simulink model "Van3"  (R2024b)
settings: Solver=ode3  StartTime=0.0  StopTime=10  FixedStep=0.001  RelTol=1e-3
Description:
  | 自适应控制
settings Model: PacingRate=1000  Creator=繁星  LastModifiedBy=14422
settings SolverCC: ShapePreserveControl=EnableAll  ZeroCrossAlgorithm=Adaptive  EnableFixedStepZeroCrossing=on
settings DataIOCC: ReturnWorkspaceOutputs=off
settings OptimizationCC: ReuseModelBlockBuffer=off
settings ModelReferenceCC: EnableRefExpFcnMdlSchedulingChecks=on
settings RTWCC: GPUComputeCapability=3.5

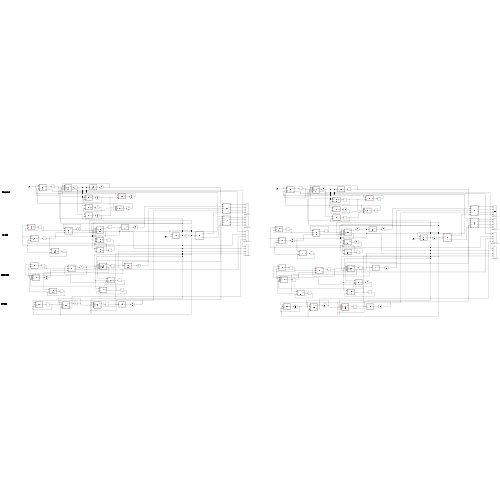
[thumbnail: Simulink's stored preview of the top-level diagram]
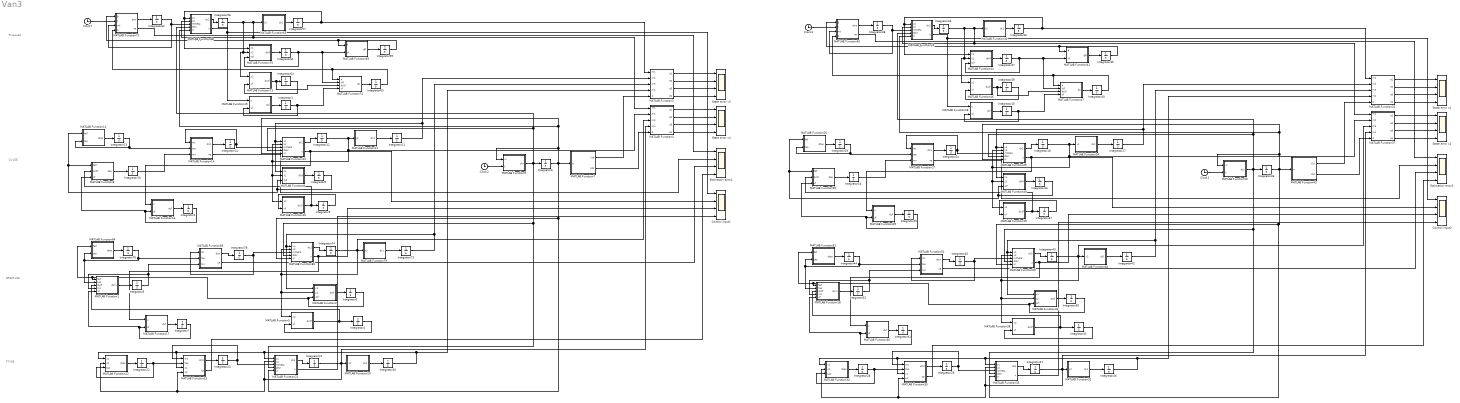
== system Van3 ==
  note: DREM-LSE
  note: CL-LSE
  note: FT-lSE
  note: Proposed
  Clock{1..3,7} (4 alike) : Clock
  Control input1 : Scope  NumInputPorts=4
  Control input2 : Scope  NumInputPorts=4
  Estimation error1 : Scope  NumInputPorts=4
  Estimation error2 : Scope  NumInputPorts=4
  Integrator{1..4,7..9,12,15,21,25,30,37..38,40..41,46,58,61..62,64..65,74} (23 alike) : Integrator
  Integrator{5,10,16,32} (4 alike) : Integrator  InitialCondition=[0;0;0]
  Integrator{11,20,57,73} (4 alike) : Integrator  InitialCondition=1
  Integrator{13,19,22,44,76} (5 alike) : Integrator  InitialCondition=1000*eye(3)
  Integrator{14,23..24,29,45,78} (6 alike) : Integrator  InitialCondition=[0.5;-1;1]*0
  Integrator{17,26,33,42} (4 alike) : Integrator  InitialCondition=0.8
  Integrator{18,27,34,43} (4 alike) : Integrator  InitialCondition=-0.5
  Integrator28 : Integrator  InitialCondition=1000*eye(3)  UpperSaturationLimit=1000  LowerSaturationLimit=0
  Integrator31 : Integrator  InitialCondition=-5
  Integrator35 : Integrator  InitialCondition=[1 0 0;0 1 0;0 0 1]*1e-7
  Integrator36 : Integrator  InitialCondition=[1;0]
  Integrator39 : Integrator  InitialCondition=-5
  Integrator47 : Integrator  InitialCondition=-5
  Integrator59 : Integrator  InitialCondition=[1 0 0;0 1 0;0 0 1]*1e-7
  Integrator6 : Integrator  InitialCondition=[1;0]
  MATLAB Function1 : MATLAB Function  TreatAsAtomicUnit=on
  MATLAB Function10 : MATLAB Function  TreatAsAtomicUnit=on
  MATLAB Function11 : MATLAB Function  TreatAsAtomicUnit=on
  MATLAB Function12 : MATLAB Function  TreatAsAtomicUnit=on
  MATLAB Function13 : MATLAB Function  TreatAsAtomicUnit=on
  MATLAB Function14 : MATLAB Function  TreatAsAtomicUnit=on
  MATLAB Function15 : MATLAB Function  TreatAsAtomicUnit=on
  MATLAB Function16 : MATLAB Function  TreatAsAtomicUnit=on
  MATLAB Function17 : MATLAB Function  TreatAsAtomicUnit=on
  MATLAB Function18 : MATLAB Function  TreatAsAtomicUnit=on
  MATLAB Function19 : MATLAB Function  TreatAsAtomicUnit=on
  MATLAB Function2 : MATLAB Function  TreatAsAtomicUnit=on
  MATLAB Function20 : MATLAB Function  TreatAsAtomicUnit=on
  MATLAB Function21 : MATLAB Function  TreatAsAtomicUnit=on
  MATLAB Function22 : MATLAB Function  TreatAsAtomicUnit=on
  MATLAB Function23 : MATLAB Function  TreatAsAtomicUnit=on
  MATLAB Function24 : MATLAB Function  TreatAsAtomicUnit=on
  MATLAB Function25 : MATLAB Function  TreatAsAtomicUnit=on
  MATLAB Function26 : MATLAB Function  TreatAsAtomicUnit=on
  MATLAB Function27 : MATLAB Function  TreatAsAtomicUnit=on
  MATLAB Function28 : MATLAB Function  TreatAsAtomicUnit=on
  MATLAB Function29 : MATLAB Function  TreatAsAtomicUnit=on
  MATLAB Function3 : MATLAB Function  TreatAsAtomicUnit=on
  MATLAB Function30 : MATLAB Function  TreatAsAtomicUnit=on
  MATLAB Function31 : MATLAB Function  TreatAsAtomicUnit=on
  MATLAB Function32 : MATLAB Function  TreatAsAtomicUnit=on
  MATLAB Function33 : MATLAB Function  TreatAsAtomicUnit=on
  MATLAB Function34 : MATLAB Function  TreatAsAtomicUnit=on
  MATLAB Function35 : MATLAB Function  TreatAsAtomicUnit=on
  MATLAB Function36 : MATLAB Function  TreatAsAtomicUnit=on
  MATLAB Function37 : MATLAB Function  TreatAsAtomicUnit=on
  MATLAB Function38 : MATLAB Function  TreatAsAtomicUnit=on
  MATLAB Function39 : MATLAB Function  TreatAsAtomicUnit=on
  MATLAB Function4 : MATLAB Function  TreatAsAtomicUnit=on
  MATLAB Function40 : MATLAB Function  TreatAsAtomicUnit=on
  MATLAB Function41 : MATLAB Function  TreatAsAtomicUnit=on
  MATLAB Function42 : MATLAB Function  TreatAsAtomicUnit=on
  MATLAB Function43 : MATLAB Function  TreatAsAtomicUnit=on
  MATLAB Function44 : MATLAB Function  TreatAsAtomicUnit=on
  MATLAB Function45 : MATLAB Function  TreatAsAtomicUnit=on
  MATLAB Function46 : MATLAB Function  TreatAsAtomicUnit=on
  MATLAB Function47 : MATLAB Function  TreatAsAtomicUnit=on
  MATLAB Function48 : MATLAB Function  TreatAsAtomicUnit=on
  MATLAB Function49 : MATLAB Function  TreatAsAtomicUnit=on
  MATLAB Function5 : MATLAB Function  TreatAsAtomicUnit=on
  MATLAB Function50 : MATLAB Function  TreatAsAtomicUnit=on
  MATLAB Function51 : MATLAB Function  TreatAsAtomicUnit=on
  MATLAB Function52 : MATLAB Function  TreatAsAtomicUnit=on
  MATLAB Function53 : MATLAB Function  TreatAsAtomicUnit=on
  MATLAB Function6 : MATLAB Function  TreatAsAtomicUnit=on
  MATLAB Function65 : MATLAB Function  TreatAsAtomicUnit=on
  MATLAB Function68 : MATLAB Function  TreatAsAtomicUnit=on
  MATLAB Function69 : MATLAB Function  TreatAsAtomicUnit=on
  MATLAB Function7 : MATLAB Function  TreatAsAtomicUnit=on
  MATLAB Function70 : MATLAB Function  TreatAsAtomicUnit=on
  MATLAB Function72 : MATLAB Function  TreatAsAtomicUnit=on
  MATLAB Function73 : MATLAB Function  TreatAsAtomicUnit=on
  MATLAB Function74 : MATLAB Function  TreatAsAtomicUnit=on
  MATLAB Function79 : MATLAB Function  TreatAsAtomicUnit=on
  MATLAB Function8 : MATLAB Function  TreatAsAtomicUnit=on
  MATLAB Function80 : MATLAB Function  TreatAsAtomicUnit=on
  MATLAB Function84 : MATLAB Function  TreatAsAtomicUnit=on
  MATLAB Function85 : MATLAB Function  TreatAsAtomicUnit=on
  MATLAB Function9 : MATLAB Function  TreatAsAtomicUnit=on
  State error x{1..4} (4 alike) : Scope  NumInputPorts=4
  wires:
  MATLAB Function73/1(dx2f) -> MATLAB Function74/3(dx2f), Integrator64/1
  MATLAB Function80/1(dx2) -> Integrator74/1
  MATLAB Function79/1(dx1) -> Integrator73/1
  MATLAB Function84/1(dtao) -> Integrator76/1
  Integrator78/1 -> MATLAB Function85/1(mt), MATLAB Function80/3(mtheta)
  Integrator62/1 -> MATLAB Function68/3(mtheta), MATLAB Function72/3(mt)
  Integrator76/1 -> MATLAB Function1/2(tao), MATLAB Function84/2(tao), MATLAB Function85/2(tao)
  MATLAB Function85/1(dmt) -> Integrator78/1
  MATLAB Function69/1(dff) -> Integrator59/1
  Integrator59/1 -> MATLAB Function72/1(B), MATLAB Function69/1(ff)
  MATLAB Function68/1(dx2) -> Integrator58/1
  MATLAB Function70/1(dWf) -> Integrator61/1
  Integrator61/1 -> MATLAB Function70/3(Wf), MATLAB Function74/2(Wf), MATLAB Function69/2(yf)
  MATLAB Function74/1(dA) -> Integrator65/1
  Integrator65/1 -> MATLAB Function72/4(A), MATLAB Function74/1(A)
  MATLAB Function65/1(dx1) -> Integrator57/1
  Integrator64/1 -> MATLAB Function73/2(xf)
  MATLAB Function72/1(dmt) -> Integrator62/1
  Clock7/1 -> MATLAB Function72/2(t)
  Integrator58/1 -> MATLAB Function68/2(x2), MATLAB Function4/1(m1), MATLAB Function65/1(x2), MATLAB Function70/2(x2), MATLAB Function73/1(x2)
  MATLAB Function3/1(dWf) -> Integrator3/1
  Integrator4/1 -> MATLAB Function5/2(xf)
  MATLAB Function5/1(dx2f) -> MATLAB Function1/3(dx2f), Integrator4/1
  Integrator3/1 -> MATLAB Function84/1(faif), MATLAB Function1/1(faif), MATLAB Function3/3(Wf)
  MATLAB Function1/1(dmn) -> Integrator5/1
  Integrator5/1 -> MATLAB Function1/4(mn), MATLAB Function85/3(mn)
  Integrator74/1 -> MATLAB Function4/3(m3), MATLAB Function5/1(x2), MATLAB Function3/2(x2), MATLAB Function80/2(x2), MATLAB Function79/1(x2)
  Integrator9/1 -> MATLAB Function10/2(xf)
  MATLAB Function8/1(dWf) -> Integrator8/1
  MATLAB Function6/1(dep) -> Integrator10/1
  MATLAB Function10/1(dx2f) -> Integrator9/1, MATLAB Function6/2(dx2f)
  Integrator14/1 -> MATLAB Function14/1(mt), MATLAB Function12/3(mtheta)
  MATLAB Function11/1(dx1) -> Integrator11/1
  MATLAB Function14/1(dmt) -> Integrator14/1
  Integrator12/1 -> MATLAB Function10/1(x2), MATLAB Function8/2(x2), MATLAB Function12/2(x2), MATLAB Function4/2(m2), MATLAB Function11/1(x2)
  MATLAB Function13/1(dtao) -> Integrator13/1
  Integrator8/1 -> MATLAB Function8/3(Wf), MATLAB Function13/1(faif), MATLAB Function6/1(faif)
  MATLAB Function12/1(dx2) -> Integrator12/1
  Integrator10/1 -> MATLAB Function14/3(mn)
  Integrator22/1 -> MATLAB Function22/3(tao), MATLAB Function23/2(tao)
  Integrator23/1 -> MATLAB Function21/3(mtheta), MATLAB Function23/1(mt)
  MATLAB Function20/1(dx1) -> Integrator20/1
  MATLAB Function23/1(dmt) -> Integrator23/1
  Integrator21/1 -> MATLAB Function4/4(m4), MATLAB Function20/1(x2), MATLAB Function23/4(x2), MATLAB Function22/2(x2), MATLAB Function21/2(x2)
  MATLAB Function22/1(dtao) -> Integrator22/1
  MATLAB Function21/1(dx2) -> Integrator21/1
  Integrator13/1 -> MATLAB Function14/2(tao), MATLAB Function13/2(tao)
  Integrator57/1 -> MATLAB Function70/1(x1), MATLAB Function68/1(x1), MATLAB Function2/1(m1)
  Integrator11/1 -> MATLAB Function2/2(m2), MATLAB Function8/1(x1), MATLAB Function12/1(x1)
  Integrator73/1 -> MATLAB Function2/3(m3), MATLAB Function3/1(x1), MATLAB Function80/1(x1)
  Integrator20/1 -> MATLAB Function22/1(x1), MATLAB Function23/3(x1), MATLAB Function21/1(x1), MATLAB Function2/4(m4)
  MATLAB Function2/2(e2) -> State error x3/2
  MATLAB Function4/1(e1) -> State error x4/1
  MATLAB Function4/2(e2) -> State error x4/2
  MATLAB Function4/4(e4) -> State error x4/4
  MATLAB Function4/3(e3) -> State error x4/3
  MATLAB Function2/3(e3) -> State error x3/3
  MATLAB Function2/4(e4) -> State error x3/4
  MATLAB Function2/1(e1) -> State error x3/1
  Clock2/1 -> MATLAB Function9/2(t)
  Integrator6/1 -> MATLAB Function21/5(xr), MATLAB Function80/5(xr), MATLAB Function12/5(xr), MATLAB Function68/5(xr), MATLAB Function9/1(xr), MATLAB Function7/1(xr)
  MATLAB Function9/1(dxr) -> MATLAB Function80/4(ddxr), MATLAB Function21/4(ddxr), MATLAB Function12/4(ddxr), MATLAB Function68/4(ddxr), Integrator6/1
  MATLAB Function7/1(x1d) -> MATLAB Function2/5(d)
  MATLAB Function7/2(x2d) -> MATLAB Function4/5(d)
  MATLAB Function72/2(ne) -> Estimation error1/1
  MATLAB Function14/2(ne) -> Estimation error1/2
  MATLAB Function85/2(ne) -> Estimation error1/3
  MATLAB Function23/2(ne) -> Estimation error1/4
  MATLAB Function21/2(u) -> Control input1/4
  MATLAB Function80/2(u) -> MATLAB Function17/1(u), Control input1/3
  MATLAB Function12/2(u) -> MATLAB Function16/1(u), Control input1/2
  MATLAB Function68/2(u) -> MATLAB Function15/1(u), Control input1/1
  MATLAB Function15/1(duf) -> Integrator1/1
  Integrator1/1 -> MATLAB Function74/4(uf), MATLAB Function15/2(uf)
  MATLAB Function16/1(duf) -> Integrator2/1
  Integrator2/1 -> MATLAB Function6/3(uf), MATLAB Function16/2(uf)
  Integrator7/1 -> MATLAB Function1/5(uf), MATLAB Function17/2(uf)
  MATLAB Function17/1(duf) -> Integrator7/1
  MATLAB Function31/4(e4) -> State error x1/4
  MATLAB Function31/1(e1) -> State error x1/1
  MATLAB Function37/3(e3) -> State error x2/3
  MATLAB Function37/1(e1) -> State error x2/1
  MATLAB Function31/2(e2) -> State error x1/2
  Integrator15/1 -> MATLAB Function47/4(uf), MATLAB Function28/2(uf)
  MATLAB Function37/2(e2) -> State error x2/2
  MATLAB Function36/1(dWf) -> Integrator30/1
  MATLAB Function40/1(dx1) -> Integrator33/1
  MATLAB Function49/1(dWf) -> Integrator46/1
  MATLAB Function50/1(dx2) -> Integrator43/1
  Integrator32/1 -> MATLAB Function18/4(mn), MATLAB Function52/3(mn)
  MATLAB Function51/1(dtao) -> Integrator44/1
  MATLAB Function44/1(dWf) -> Integrator37/1
  Integrator19/1 -> MATLAB Function27/2(tao), MATLAB Function26/2(tao)
  Integrator28/1 -> MATLAB Function34/3(tao), MATLAB Function35/2(tao)
  Integrator37/1 -> MATLAB Function44/3(Wf), MATLAB Function47/2(Wf), MATLAB Function42/2(yf)
  MATLAB Function18/1(dmn) -> Integrator32/1
  MATLAB Function39/1(dep) -> Integrator16/1
  MATLAB Function26/1(dtao) -> Integrator19/1
  MATLAB Function35/1(dmt) -> Integrator29/1
  Clock3/1 -> MATLAB Function45/2(t)
  MATLAB Function33/1(dx2) -> Integrator27/1
  Integrator44/1 -> MATLAB Function18/2(tao), MATLAB Function51/2(tao), MATLAB Function52/2(tao)
  MATLAB Function19/1(dx2f) -> Integrator47/1, MATLAB Function39/2(dx2f)
  Integrator40/1 -> MATLAB Function45/4(A), MATLAB Function47/1(A)
  Integrator16/1 -> MATLAB Function27/3(mn)
  MATLAB Function42/1(dff) -> Integrator35/1
  MATLAB Function31/3(e3) -> State error x1/3
  Integrator24/1 -> MATLAB Function27/1(mt), MATLAB Function25/3(mtheta)
  MATLAB Function41/1(dx2) -> Integrator34/1
  Integrator34/1 -> MATLAB Function41/2(x2), MATLAB Function37/1(m1), MATLAB Function40/1(x2), MATLAB Function44/2(x2), MATLAB Function46/1(x2)
  MATLAB Function41/2(u) -> MATLAB Function28/1(u), Control input2/1
  MATLAB Function53/1(dxr) -> MATLAB Function50/4(ddxr), MATLAB Function33/4(ddxr), MATLAB Function25/4(ddxr), MATLAB Function41/4(ddxr), Integrator36/1
  Integrator36/1 -> MATLAB Function33/5(xr), MATLAB Function50/5(xr), MATLAB Function25/5(xr), MATLAB Function41/5(xr), MATLAB Function53/1(xr), MATLAB Function43/1(xr)
  Clock1/1 -> MATLAB Function53/2(t)
  Integrator26/1 -> MATLAB Function34/1(x1), MATLAB Function35/3(x1), MATLAB Function33/1(x1), MATLAB Function31/4(m4)
  Integrator17/1 -> MATLAB Function31/2(m2), MATLAB Function49/1(x1), MATLAB Function25/1(x1)
  Integrator27/1 -> MATLAB Function37/4(m4), MATLAB Function32/1(x2), MATLAB Function34/2(x2), MATLAB Function35/4(x2), MATLAB Function33/2(x2)
  MATLAB Function29/1(duf) -> Integrator25/1
  Integrator25/1 -> MATLAB Function39/3(uf), MATLAB Function29/2(uf)
  MATLAB Function52/2(ne) -> Estimation error2/3
  MATLAB Function45/2(ne) -> Estimation error2/1
  MATLAB Function30/1(duf) -> Integrator41/1
  MATLAB Function27/2(ne) -> Estimation error2/2
  Integrator41/1 -> MATLAB Function18/5(uf), MATLAB Function30/2(uf)
  Integrator33/1 -> MATLAB Function44/1(x1), MATLAB Function41/1(x1), MATLAB Function31/1(m1)
  Integrator43/1 -> MATLAB Function37/3(m3), MATLAB Function38/1(x2), MATLAB Function36/2(x2), MATLAB Function50/2(x2), MATLAB Function48/1(x2)
  MATLAB Function35/2(ne) -> Estimation error2/4
  Integrator38/1 -> MATLAB Function41/3(mtheta), MATLAB Function45/3(mt)
  MATLAB Function46/1(dx2f) -> MATLAB Function47/3(dx2f), Integrator39/1
  MATLAB Function43/2(x2d) -> MATLAB Function37/5(d)
  MATLAB Function32/1(dx1) -> Integrator26/1
  MATLAB Function28/1(duf) -> Integrator15/1
  MATLAB Function43/1(x1d) -> MATLAB Function31/5(d)
  MATLAB Function25/1(dx2) -> Integrator18/1
  MATLAB Function37/4(e4) -> State error x2/4
  Integrator42/1 -> MATLAB Function31/3(m3), MATLAB Function36/1(x1), MATLAB Function50/1(x1)
  Integrator47/1 -> MATLAB Function19/2(xf)
  Integrator29/1 -> MATLAB Function33/3(mtheta), MATLAB Function35/1(mt)
  Integrator31/1 -> MATLAB Function38/2(xf)
  Integrator35/1 -> MATLAB Function45/1(B), MATLAB Function42/1(ff)
  MATLAB Function52/1(dmt) -> Integrator45/1
  MATLAB Function27/1(dmt) -> Integrator24/1
  Integrator30/1 -> MATLAB Function51/1(faif), MATLAB Function18/1(faif), MATLAB Function36/3(Wf)
  MATLAB Function47/1(dA) -> Integrator40/1
  Integrator39/1 -> MATLAB Function46/2(xf)
  MATLAB Function38/1(dx2f) -> MATLAB Function18/3(dx2f), Integrator31/1
  Integrator45/1 -> MATLAB Function52/1(mt), MATLAB Function50/3(mtheta)
  MATLAB Function45/1(dmt) -> Integrator38/1
  MATLAB Function33/2(u) -> Control input2/4
  MATLAB Function48/1(dx1) -> Integrator42/1
  Integrator46/1 -> MATLAB Function49/3(Wf), MATLAB Function26/1(faif), MATLAB Function39/1(faif)
  Integrator18/1 -> MATLAB Function19/1(x2), MATLAB Function49/2(x2), MATLAB Function25/2(x2), MATLAB Function37/2(m2), MATLAB Function24/1(x2)
  MATLAB Function24/1(dx1) -> Integrator17/1
  MATLAB Function50/2(u) -> MATLAB Function30/1(u), Control input2/3
  MATLAB Function25/2(u) -> MATLAB Function29/1(u), Control input2/2
  MATLAB Function34/1(dtao) -> Integrator28/1

== matlab function Van3/MATLAB Function14 ==
  data: dmt output size=3,1; mt input; tao input; mn input; ne output
function [dmt,ne]   = fcn(mt,tao,mn)



theta=[0.5;-1;1];

Q=inv(tao)-inv(1000*eye(3));

gama=100;

ne=norm(theta-mt);
dmt=gama*tao*(mn-Q*mt);

== matlab function Van3/MATLAB Function6 ==
  data: faif input; dep output; dx2f input; uf input
function dep = fcn(faif,dx2f,uf)



dep=faif'*(dx2f-uf);

== matlab function Van3/MATLAB Function2 ==
  data: m1 input; e1 output; m2 input; m3 input; e2 output; e3 output; m4 input; e4 output; d input
function [e1,e2,e3,e4]  = fcn(m1,m2,m3,m4,d)



e1=norm(m1-d);
e2=norm(m2-d);
e3=norm(m3-d);
e4=norm(m4-d);
e1=norm(m1-d);
e2=norm(m2-d);
e3=norm(m3-d);
e4=norm(m4-d);

== matlab function Van3/MATLAB Function8 ==
  data: x1 input; dWf output; x2 input; Wf input
function dWf  = fcn(x1,x2,Wf)

A=[-x1,x2,-x1*x1*x2];
dWf=-0.1*Wf+A;

== matlab function Van3/MATLAB Function15 ==
  data: u input; uf input; duf output
function duf  = fcn(u,uf)


duf=-0.1*uf+u;

== matlab function Van3/MATLAB Function16 ==
  data: u input; uf input; duf output
function duf  = fcn(u,uf)


duf=-0.1*uf+u;

== matlab function Van3/MATLAB Function17 ==
  data: u input; uf input; duf output
function duf  = fcn(u,uf)


duf=-0.1*uf+u;

== matlab function Van3/MATLAB Function4 ==
  data: m1 input; e1 output; m2 input; m3 input; e2 output; e3 output; m4 input; e4 output; d input
function [e1,e2,e3,e4]  = fcn(m1,m2,m3,m4,d)



e1=norm(m1-d);
e2=norm(m2-d);
e3=norm(m3-d);
e4=norm(m4-d);
e1=norm(m1-d);
e2=norm(m2-d);
e3=norm(m3-d);
e4=norm(m4-d);

== matlab function Van3/MATLAB Function18 ==
  data: faif input; dmn output; tao input; dx2f input; mn input; uf input
function dmn = fcn(faif,tao,dx2f,mn,uf)



dmn=tao*faif'*(dx2f-uf-faif*mn);

== matlab function Van3/MATLAB Function19 ==
  data: x2 input; xf input; dx2f output
function dx2f  = fcn(x2,xf)


dx2f=-0.1*xf+x2;

== matlab function Van3/MATLAB Function20 ==
  data: x2 input; dx1 output
function dx1 = fcn(x2)
dx1=x2;

== matlab function Van3/MATLAB Function21 ==
  data: x1 input; x2 input; dx2 output; mtheta input; ddxr input; xr input; u output
function [dx2,u] = fcn(x1,x2,mtheta,ddxr,xr)


%unknown parameter vector
theta=[0.5;-1;1];

x=[x1;x2];


u=ddxr(2)-[4 4]*(x-xr)-[-x1,x2,-x1*x1*x2]*mtheta;


dx2=[-x1,x2,-x1*x1*x2]*theta+u;

== matlab function Van3/MATLAB Function22 ==
  data: x1 input; x2 input; dtao output; tao input
function dtao = fcn(x1,x2,tao)


fai=[-x1,x2,-x1*x1*x2];

dtao=-tao*fai'*fai*tao;

== matlab function Van3/MATLAB Function23 ==
  data: dmt output size=3,1; mt input; ne output; tao input; x1 input; x2 input
function [dmt,ne]   = fcn(mt,tao,x1,x2)



theta=[0.5;-1;1];
fai=[-x1,x2,-x1*x1*x2];


  ne=norm(theta-mt);


dmt=tao*fai'*fai*(theta-mt);

== matlab function Van3/MATLAB Function24 ==
  data: x2 input; dx1 output
function dx1 = fcn(x2)
dx1=x2;

== matlab function Van3/MATLAB Function25 ==
  data: x1 input; x2 input; dx2 output; mtheta input; ddxr input; xr input; u output
function [dx2,u] = fcn(x1,x2,mtheta,ddxr,xr)


%unknown parameter vector
theta=[0.5;-1;1];
theta=[2;-2;3];
theta=[2;-2;3]*2;

x=[x1;x2];


u=ddxr(2)-[4 4]*(x-xr)-[-x1,x2,-x1*x1*x2]*mtheta;


dx2=[-x1,x2,-x1*x1*x2]*theta+u;

== matlab function Van3/MATLAB Function1 ==
  data: faif input; dmn output; tao input; dx2f input; mn input; uf input
function dmn = fcn(faif,tao,dx2f,mn,uf)



dmn=tao*faif'*(dx2f-uf-faif*mn);

== matlab function Van3/MATLAB Function26 ==
  data: faif input; dtao output; tao input
function dtao = fcn(faif,tao)


dtao=-tao*faif'*faif*tao;

== matlab function Van3/MATLAB Function27 ==
  data: dmt output size=3,1; mt input; tao input; mn input; ne output
function [dmt,ne]   = fcn(mt,tao,mn)



theta=[0.5;-1;1];
theta=[2;-2;3];
theta=[2;-2;3]*2;

Q=inv(tao)-inv(1000*eye(3));

gama=100;

ne=norm(theta-mt);
dmt=gama*tao*(mn-Q*mt);

== matlab function Van3/MATLAB Function28 ==
  data: u input; uf input; duf output
function duf  = fcn(u,uf)


duf=-0.1*uf+u;

== matlab function Van3/MATLAB Function29 ==
  data: u input; uf input; duf output
function duf  = fcn(u,uf)


duf=-0.1*uf+u;

== matlab function Van3/MATLAB Function30 ==
  data: u input; uf input; duf output
function duf  = fcn(u,uf)


duf=-0.1*uf+u;

== matlab function Van3/MATLAB Function31 ==
  data: m1 input; e1 output; m2 input; m3 input; e2 output; e3 output; m4 input; e4 output; d input
function [e1,e2,e3,e4]  = fcn(m1,m2,m3,m4,d)



e1=norm(m1-d);
e2=norm(m2-d);
e3=norm(m3-d);
e4=norm(m4-d);

== matlab function Van3/MATLAB Function32 ==
  data: x2 input; dx1 output
function dx1 = fcn(x2)
dx1=x2;

== matlab function Van3/MATLAB Function33 ==
  data: x1 input; x2 input; dx2 output; mtheta input; ddxr input; xr input; u output
function [dx2,u] = fcn(x1,x2,mtheta,ddxr,xr)


%unknown parameter vector
theta=[0.5;-1;1];
theta=[2;-2;3];
theta=[2;-2;3]*2;

x=[x1;x2];


u=ddxr(2)-[4 4]*(x-xr)-[-x1,x2,-x1*x1*x2]*mtheta;


dx2=[-x1,x2,-x1*x1*x2]*theta+u;

== matlab function Van3/MATLAB Function34 ==
  data: x1 input; x2 input; dtao output; tao input
function dtao = fcn(x1,x2,tao)


fai=[-x1,x2,-x1*x1*x2];

dtao=-tao*fai'*fai*tao;

== matlab function Van3/MATLAB Function35 ==
  data: dmt output size=3,1; mt input; ne output; tao input; x1 input; x2 input
function [dmt,ne]   = fcn(mt,tao,x1,x2)



theta=[0.5;-1;1];
theta=[2;-2;3];
theta=[2;-2;3]*2;
fai=[-x1,x2,-x1*x1*x2];


  ne=norm(theta-mt);


dmt=tao*fai'*fai*(theta-mt);

== matlab function Van3/MATLAB Function36 ==
  data: x1 input; dWf output; x2 input; Wf input
function dWf  = fcn(x1,x2,Wf)

A=[-x1,x2,-x1*x1*x2];
dWf=-0.1*Wf+A;

== matlab function Van3/MATLAB Function37 ==
  data: m1 input; e1 output; m2 input; m3 input; e2 output; e3 output; m4 input; e4 output; d input
function [e1,e2,e3,e4]  = fcn(m1,m2,m3,m4,d)



e1=norm(m1-d);
e2=norm(m2-d);
e3=norm(m3-d);
e4=norm(m4-d);

== matlab function Van3/MATLAB Function7 ==
  data: x1d output size=1; xr input double; x2d output size=1
function [x1d,x2d]  = fcn(xr)



x1d=xr(1);
x2d=xr(2);

== matlab function Van3/MATLAB Function38 ==
  data: x2 input; xf input; dx2f output
function dx2f  = fcn(x2,xf)


dx2f=-0.1*xf+x2;

== matlab function Van3/MATLAB Function39 ==
  data: faif input; dep output; dx2f input; uf input
function dep = fcn(faif,dx2f,uf)



dep=faif'*(dx2f-uf);

== matlab function Van3/MATLAB Function40 ==
  data: x2 input; dx1 output
function dx1 = fcn(x2)
dx1=x2;

== matlab function Van3/MATLAB Function41 ==
  data: x1 input; x2 input size=1; dx2 output size=1; mtheta input; ddxr input; xr input; u output
function [dx2,u] = fcn(x1,x2,mtheta,ddxr,xr)


%unknown parameter vector
theta=[0.5;-1;1];
theta=[2;-2;3]*2;

x=[x1;x2];


u=ddxr(2)-[4 4]*(x-xr)-[-x1,x2,-x1*x1*x2]*mtheta;


dx2=[-x1,x2,-x1*x1*x2]*theta+u;

== matlab function Van3/MATLAB Function42 ==
  data: ff input; dff output; yf input
function dff = fcn(ff,yf)


dff=-1*ff+yf'*yf;

== matlab function Van3/MATLAB Function43 ==
  data: x1d output size=1; xr input double; x2d output size=1
function [x1d,x2d]  = fcn(xr)



x1d=xr(1);
x2d=xr(2);

== matlab function Van3/MATLAB Function44 ==
  data: x1 input; dWf output; x2 input; Wf input
function dWf  = fcn(x1,x2,Wf)

A=[-x1,x2,-x1*x1*x2];
dWf=-0.1*Wf+A;

== matlab function Van3/MATLAB Function45 ==
  data: B input; dmt output size=3,1; t input; mt input; A input size=3,1; ne output
function [dmt,ne]    = fcn(B,t,mt,A)





theta=[0.5;-1;1];
theta=[2;-2;3]*2;
k1=1e-7;

  ne=norm(theta-mt);

 k=0.2;

ee=B\A-(1*eye(3)-k1*eye(3)*exp(-1*t)/B)*mt;

dmt=exp(abs(ee).^k).*sign(ee).*abs(ee).^(1-k)/(k*2);

== matlab function Van3/MATLAB Function3 ==
  data: x1 input; dWf output; x2 input; Wf input
function dWf  = fcn(x1,x2,Wf)

A=[-x1,x2,-x1*x1*x2];
dWf=-0.1*Wf+A;

== matlab function Van3/MATLAB Function46 ==
  data: x2 input; xf input; dx2f output
function dx2f  = fcn(x2,xf)


dx2f=-0.1*xf+x2;

== matlab function Van3/MATLAB Function47 ==
  data: A input; dA output; Wf input; dx2f input; uf input
function dA  = fcn(A,Wf,dx2f,uf)

theta=[0.5;-1;1];
dA=-1*A+Wf'*(dx2f-uf);
% dA=-1*A+Wf'*Wf*theta;

== matlab function Van3/MATLAB Function48 ==
  data: x2 input; dx1 output
function dx1 = fcn(x2)
dx1=x2;

== matlab function Van3/MATLAB Function49 ==
  data: x1 input; dWf output; x2 input; Wf input
function dWf  = fcn(x1,x2,Wf)

A=[-x1,x2,-x1*x1*x2];
dWf=-0.1*Wf+A;

== matlab function Van3/MATLAB Function50 ==
  data: x1 input; x2 input; dx2 output; mtheta input; ddxr input; xr input; u output
function [dx2,u] = fcn(x1,x2,mtheta,ddxr,xr)


%unknown parameter vector
theta=[0.5;-1;1];
theta=[2;-2;3];
theta=[2;-2;3]*2;

x=[x1;x2];


u=ddxr(2)-[4 4]*(x-xr)-[-x1,x2,-x1*x1*x2]*mtheta;


dx2=[-x1,x2,-x1*x1*x2]*theta+u;

== matlab function Van3/MATLAB Function51 ==
  data: faif input; dtao output; tao input
function dtao = fcn(faif,tao)


dtao=-tao*faif'*faif*tao;

== matlab function Van3/MATLAB Function52 ==
  data: dmt output size=3,1; mt input; tao input; mn input; ne output
function [dmt,ne]   = fcn(mt,tao,mn)



theta=[0.5;-1;1];
theta=[2;-2;3];
theta=[2;-2;3]*2;

gama=100;

  ne=norm(theta-mt);







A=eye(3)-inv(1000*eye(3))*tao;
adj_A = zeros(3,3);

% 计算每个余因子元素（展开循环优化性能）
adj_A(1,1) =  det(A([2,3], [2,3])) * (-1)^(1+1);
adj_A(1,2) = det(A([2,3], [1,3])) * (-1)^(1+2);
adj_A(1,3) =  det(A([2,3], [1,2])) * (-1)^(1+3);

adj_A(2,1) = det(A([1,3], [2,3])) * (-1)^(2+1);
adj_A(2,2) =  det(A([1,3], [1,3])) * (-1)^(2+2);
adj_A(2,3) = det(A([1,3], [1,2])) * (-1)^(2+3);

adj_A(3,1) =  det(A([1,2], [2,3])) * (-1)^(3+1);
adj_A(3,2) = det(A([1,2], [1,3])) * (-1)^(3+2);
adj_A(3,3) =  det(A([1,2], [1,2])) * (-1)^(3+3);

% 转置余因子矩阵得到伴随矩阵
adjoint1 = adj_A';



fai=adjoint1*mn;
deta=det(eye(3)-inv(1000*eye(3))*tao);
dmt=gama*deta*(fai-deta*mt);

== matlab function Van3/MATLAB Function53 ==
  data: xr input; dxr output; t input
function dxr = fcn(xr,t)


if t<=5
    r=0;
else
r=0.5;
end
dxr=[0 1;-4 -4]*xr+[0;4]*r;

== matlab function Van3/MATLAB Function65 ==
  data: x2 input; dx1 output
function dx1 = fcn(x2)
dx1=x2;

== matlab function Van3/MATLAB Function68 ==
  data: x1 input; x2 input size=1; dx2 output size=1; mtheta input; ddxr input; xr input; u output
function [dx2,u] = fcn(x1,x2,mtheta,ddxr,xr)


%unknown parameter vector
theta=[0.5;-1;1];

x=[x1;x2];


u=ddxr(2)-[4 4]*(x-xr)-[-x1,x2,-x1*x1*x2]*mtheta;


dx2=[-x1,x2,-x1*x1*x2]*theta+u;

== matlab function Van3/MATLAB Function9 ==
  data: xr input; dxr output; t input
function dxr = fcn(xr,t)


if t<=5
    r=0;
else
r=0.5;
end
dxr=[0 1;-4 -4]*xr+[0;4]*r;

== matlab function Van3/MATLAB Function69 ==
  data: ff input; dff output; yf input
function dff = fcn(ff,yf)


dff=-1*ff+yf'*yf;

== matlab function Van3/MATLAB Function70 ==
  data: x1 input; dWf output; x2 input; Wf input
function dWf  = fcn(x1,x2,Wf)

A=[-x1,x2,-x1*x1*x2];
dWf=-0.1*Wf+A;

== matlab function Van3/MATLAB Function72 ==
  data: B input; dmt output size=3,1; t input; mt input; A input size=3,1; ne output
function [dmt,ne]    = fcn(B,t,mt,A)





theta=[0.5;-1;1];
k1=1e-7;

  ne=norm(theta-mt);

 k=0.2;

ee=B\A-(1*eye(3)-k1*eye(3)*exp(-1*t)/B)*mt;

dmt=exp(abs(ee).^k).*sign(ee).*abs(ee).^(1-k)/(k*2);

== matlab function Van3/MATLAB Function73 ==
  data: x2 input; xf input; dx2f output
function dx2f  = fcn(x2,xf)


dx2f=-0.1*xf+x2;

== matlab function Van3/MATLAB Function74 ==
  data: A input; dA output; Wf input; dx2f input; uf input
function dA  = fcn(A,Wf,dx2f,uf)

theta=[0.5;-1;1];
dA=-1*A+Wf'*(dx2f-uf);
% dA=-1*A+Wf'*Wf*theta;

== matlab function Van3/MATLAB Function79 ==
  data: x2 input; dx1 output
function dx1 = fcn(x2)
dx1=x2;

== matlab function Van3/MATLAB Function80 ==
  data: x1 input; x2 input; dx2 output; mtheta input; ddxr input; xr input; u output
function [dx2,u] = fcn(x1,x2,mtheta,ddxr,xr)


%unknown parameter vector
theta=[0.5;-1;1];

x=[x1;x2];


u=ddxr(2)-[4 4]*(x-xr)-[-x1,x2,-x1*x1*x2]*mtheta;


dx2=[-x1,x2,-x1*x1*x2]*theta+u;

== matlab function Van3/MATLAB Function84 ==
  data: faif input; dtao output; tao input
function dtao = fcn(faif,tao)


dtao=-tao*faif'*faif*tao;

== matlab function Van3/MATLAB Function85 ==
  data: dmt output size=3,1; mt input; tao input; mn input; ne output
function [dmt,ne]   = fcn(mt,tao,mn)



theta=[0.5;-1;1];

gama=100;

  ne=norm(theta-mt);







A=eye(3)-inv(1000*eye(3))*tao;
adj_A = zeros(3,3);

% 计算每个余因子元素（展开循环优化性能）
adj_A(1,1) =  det(A([2,3], [2,3])) * (-1)^(1+1);
adj_A(1,2) = det(A([2,3], [1,3])) * (-1)^(1+2);
adj_A(1,3) =  det(A([2,3], [1,2])) * (-1)^(1+3);

adj_A(2,1) = det(A([1,3], [2,3])) * (-1)^(2+1);
adj_A(2,2) =  det(A([1,3], [1,3])) * (-1)^(2+2);
adj_A(2,3) = det(A([1,3], [1,2])) * (-1)^(2+3);

adj_A(3,1) =  det(A([1,2], [2,3])) * (-1)^(3+1);
adj_A(3,2) = det(A([1,2], [1,3])) * (-1)^(3+2);
adj_A(3,3) =  det(A([1,2], [1,2])) * (-1)^(3+3);

% 转置余因子矩阵得到伴随矩阵
adjoint1 = adj_A';



fai=adjoint1*mn;
deta=det(eye(3)-inv(1000*eye(3))*tao);
dmt=gama*deta*(fai-deta*mt);

== matlab function Van3/MATLAB Function5 ==
  data: x2 input; xf input; dx2f output
function dx2f  = fcn(x2,xf)


dx2f=-0.1*xf+x2;

== matlab function Van3/MATLAB Function10 ==
  data: x2 input; xf input; dx2f output
function dx2f  = fcn(x2,xf)


dx2f=-0.1*xf+x2;

== matlab function Van3/MATLAB Function11 ==
  data: x2 input; dx1 output
function dx1 = fcn(x2)
dx1=x2;

== matlab function Van3/MATLAB Function12 ==
  data: x1 input; x2 input; dx2 output; mtheta input; ddxr input; xr input; u output
function [dx2,u] = fcn(x1,x2,mtheta,ddxr,xr)


%unknown parameter vector
theta=[0.5;-1;1];

x=[x1;x2];


u=ddxr(2)-[4 4]*(x-xr)-[-x1,x2,-x1*x1*x2]*mtheta;


dx2=[-x1,x2,-x1*x1*x2]*theta+u;

== matlab function Van3/MATLAB Function13 ==
  data: faif input; dtao output; tao input
function dtao = fcn(faif,tao)


dtao=-tao*faif'*faif*tao;
